simulink model "mpc_aircraft"  (R2015a)
settings: Solver=ode45  SolverMode=SingleTasking  StartTime=0.0  StopTime=10  RelTol=1e-3
values from neighbouring files (symbols this model uses):
  A = [-0.0151 -60.5651 0 -32.174 ... (first row only)    [mpcaircraft.m]
  B = [-2.516 -13.136 ... (first row only)    [mpcaircraft.m]
  C = [0 1 0 0 ... (first row only)    [mpcaircraft.m]
  D = [0 0 ... (first row only)    [mpcaircraft.m]
  p = 10    [mpcaircraft.m]
  x0 = zeros(4,1)    [mpcaircraft.m]
undefined symbols (not defined in the file or in its folder): iA, lastu, lastx, MVscale, nv, nym, Rscale, st, ts, uoff, xoff
libraries: mpcsigdimcheck_private x14
settings Model: CovSFcnEnable=off  ExtModeTrigMode=oneshot  ExtModeArmWhenConnect=off  Creator=The MathWorks Inc.  LastModifiedBy=Yi
settings OptimizationCC: BlockReduction=off  BooleanDataType=off
settings DebuggingCC: SaveWithParameterizedLinksMsg=none  UnderspecifiedInitializationDetection=Classic  MergeDetectMultiDrivingBlocksExec=none  SignalResolutionControl=TryResolveAllWithWarning
settings HardwareCC: TargetUnknown=on

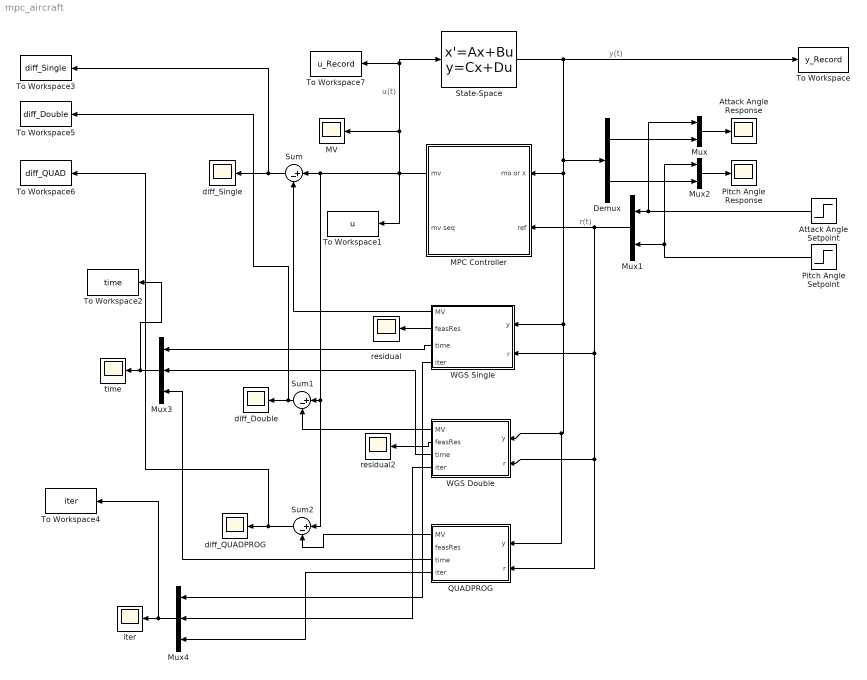
== system mpc_aircraft ==
  note: u(t)
  note: y(t)
  note: r(t)
  Attack Angle Response : Scope
      settings: TimeRange=7  YMin=-0.05  YMax=0.15  DataFormat=Structure
  Attack Angle Setpoint : Step  Time=4  After=0.1  SampleTime=0
  Demux : Demux  Outputs=2
  MPC Controller : Subsystem  AncestorBlock=mpclib/MPC Controller  InitFcn=impcblock_InitFcn  StartFcn=impcblock_StartFcn  mask(MPC){mpcobj=mpcobj, x0=[], is_multiple=0, enable_value=0, n_mv=2, n_mo=2, n_md=0, n_ts=0.05, is_designfromscratch=0, return_u0=off, ref_from_ws=off, ref_signal_name=[], ref_preview=on, md_from_ws=off, md_signal_name=[], md_preview=on, from_project=off, project_file=MPCtask.mat, project_name=, task_name=, md_inport=off, mv_inport=off, cost_outport=off, return_sequence=on, return_qpstatus=off, return_state=off, state_inport=off, lims_inport=off, ywt_inport=off, uwt_inport=off, duwt_inport=off, rhoeps_inport=off, uref_inport=off, BlockDataType=double, SampleTimeInherited=off, switch_inport=off}
      mask prompts: mpcobj "MPC:general:BlgIMPC"; x0 "MPC:general:BlgState"; is_multiple "Flag indicating the block is part of multiple blocks"; enable_value "Value enabling optimization"; n_mv "Number of MVs"; n_mo "Number of MOs"; n_md "Number of MDs"; n_ts "Sample Time"; is_designfromscratch "Design from scratch flag"; return_u0 "Export u0"; ref_from_ws "Obsolete"; ref_signal_name "Obsolete"; ref_preview "Obsolete"; md_from_ws "Obsolete"; md_signal_name "Obsolete"; md_preview "Obsolete"; from_project "Obsolete"; project_file "Obsolete"; project_name "Obsolete"; task_name "Obsolete"; md_inport "MPC:general:BlgMD"; mv_inport "MPC:general:BlgEXTMV"; cost_outport "MPC:general:BlgCOST"; return_sequence "MPC:general:BlgMVSEQ"; return_qpstatus "MPC:general:BlgQPSTATUS"; return_state "MPC:general:BlgESTSTATE"; state_inport "MPC:general:BlgXKK"; lims_inport "MPC:general:BlgLIMITS"; ywt_inport "MPC:general:BlgYWT"; uwt_inport "MPC:general:BlgUWT"; duwt_inport "MPC:general:BlgDUWT"; rhoeps_inport "MPC:general:BlgECRWT"; uref_inport "MPC:general:BlgMVTARGET"; BlockDataType "MPC:general:BlgDATATYPE"; SampleTimeInherited "MPC:general:BlgTS"; switch_inport "MPC:general:BlgSWITCH"
      mask help: MPC:utility:MaskDescMPC1
      mask init:
      | [blk,ts,A,Cm,Bu,Bv,Dvm,isQP,strmoorx,nmoorx,nu,nv,ny,nx,nym...
      |     degrees,L,M,H,Hinv,Linv,iA,Ac,Kx,Ku1,Kut,Kr,Kv,...
      |     Mlim,Mx,Mu1,Mv,z_degrees,utarget,...
      |     lastx,lastu,p,xoff,uoff,yoff,voff,myoff,no_md,no_ref,...
      |     maxiter,nxQP,openloopflag,no_ym,...
      |     lims_inport,no_umin,no_umax,no_ymin,no_ymax,...
      |     switch_inport,no_switch,enable_value,...
      |     return_cost,return_sequence,CustomEstimation,...
      |     no_ywt, no_uwt, no_duwt, no_rhoeps, no_uref, no_mv, ...
      |     Wy,Wdu,Jm,SuJm,Su1,Sx,Hv,Wu,I1,...
      |     isAdaptive, C, Dv, Mrows, nCC, Ecc, Fcc, Scc, Gcc, ...
      |     Uscale, Yscale, nxp, nxindist, mvindex, mdindex, unindex,  ...
      |     myindex,Rscale,MVscale,MDscale] = impcblock_MaskInitFcnParameter();
      | impcblock_MaskInitFcnResize(gcb,nv,nu,ny);
      settings: DeleteFcn=impcblock_DeleteFcn
      mask Help: eval('mpcCSHelp(''MPCmask'',''HelpBrowser'')');
      mask Callback state_inport: mpc_blockdialogcallback(gcb);
      mask DialogControl design_button Prompt: MPC:general:BlgDesignButton
      mask DialogControl design_button Callback: mpc_designcallback(gcbh)
      mask DialogControl review_button Prompt: MPC:general:BlgReviewButton
      mask DialogControl review_button Callback: mpc_reviewcallback(gcbh)
      mask Display:
      | fprintf('MPC');
      | port_label('output', 1, 'mv')
      | port_label('input', 1, 'mo')
      | port_label('input', 2, 'ref')
      | port_label('output', 2, 'mv.seq')
  MV : Scope
      settings: TimeRange=7  YMin=-0.05  YMax=0.15  SaveName=ScopeData11  DataFormat=Structure
  Mux : Mux  Inputs=2
  Mux1 : Mux  Inputs=2
  Mux2 : Mux  Inputs=2
  Mux3 : Mux  Inputs=3
  Mux4 : Mux  Inputs=3
  Pitch Angle Response : Scope
      settings: TimeRange=7  YMin=0  YMax=15  DataFormat=Structure
  Pitch Angle Setpoint : Step  After=10  SampleTime=0
  QUADPROG : Subsystem
  State-Space : StateSpace  A=A  B=B  C=C  D=D  X0=x0
  Sum : Sum  Inputs=|+-
  Sum1 : Sum  Inputs=|+-
  Sum2 : Sum  Inputs=|+-
  To Workspace : ToWorkspace  VariableName=y_Record  SampleTime=-1
  To Workspace1 : ToWorkspace  VariableName=u  SampleTime=-1
  To Workspace2 : ToWorkspace  VariableName=time  SampleTime=-1
  To Workspace3 : ToWorkspace  VariableName=diff_Single  SampleTime=-1
  To Workspace4 : ToWorkspace  VariableName=iter  SampleTime=-1
  To Workspace5 : ToWorkspace  VariableName=diff_Double  SampleTime=-1
  To Workspace6 : ToWorkspace  VariableName=diff_QUAD  SampleTime=-1
  To Workspace7 : ToWorkspace  VariableName=u_Record  SampleTime=-1
  WGS Double : Subsystem
  WGS Single : Subsystem
  diff_Double : Scope
      settings: TimeRange=7  YMin=-0.05  YMax=0.15  SaveName=ScopeData4  DataFormat=Structure
  diff_QUADPROG : Scope
      settings: TimeRange=7  YMin=-0.05  YMax=0.15  SaveName=ScopeData9  DataFormat=Structure
  diff_Single : Scope
      settings: TimeRange=7  YMin=-0.05  YMax=0.15  SaveName=ScopeData3  DataFormat=Structure
  iter : Scope
      settings: TimeRange=7  YMin=-0.05  YMax=0.15  SaveName=ScopeData10  DataFormat=Structure
  residual : Scope
      settings: TimeRange=7  YMin=-0.05  YMax=0.15  SaveName=ScopeData2  DataFormat=Structure
  residual2 : Scope
      settings: TimeRange=7  YMin=-0.05  YMax=0.15  SaveName=ScopeData7  DataFormat=Structure
  "time " : Scope
      settings: TimeRange=7  YMin=-0.05  YMax=0.15  SaveName=ScopeData8  DataFormat=Structure
  wires:
  State-Space/1 -> To Workspace/1, QUADPROG/1(y), WGS Double/1(y), WGS Single/1(y), MPC Controller/1(mo or x), Demux/1
  Mux/1 -> Attack Angle Response/1
  MPC Controller/1(mv) -> MV/1, To Workspace7/1, State-Space/1, Sum2/1, Sum1/1, Sum/1, To Workspace1/1
  Attack Angle Setpoint/1 -> Mux/1, Mux1/1
  Pitch Angle Setpoint/1 -> Mux2/1, Mux1/2
  Mux1/1 -> QUADPROG/2(r), WGS Double/2(r), WGS Single/2(r), MPC Controller/2(ref)
  Demux/1 -> Mux/2
  Mux2/1 -> Pitch Angle Response/1
  Demux/2 -> Mux2/2
  WGS Single/1(MV) -> Sum/2
  WGS Single/2(feasRes) -> residual/1
  WGS Double/1(MV) -> Sum1/2
  WGS Double/2(feasRes) -> residual2/1
  WGS Double/3(time) -> Mux3/2
  Mux3/1 -> To Workspace2/1, "time "/1
  QUADPROG/3(time) -> Mux3/3
  QUADPROG/1(MV) -> Sum2/2
  WGS Single/3(time) -> Mux3/1
  WGS Double/4(iter) -> Mux4/2
  Mux4/1 -> To Workspace4/1, iter/1
  QUADPROG/4(iter) -> Mux4/3
  WGS Single/4(iter) -> Mux4/1
  Sum/1 -> To Workspace3/1, diff_Single/1
  Sum1/1 -> To Workspace5/1, diff_Double/1
  Sum2/1 -> To Workspace6/1, diff_QUADPROG/1

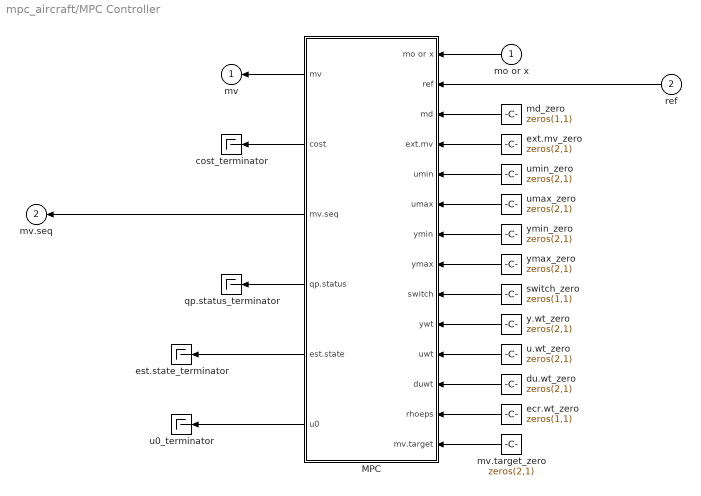
== system mpc_aircraft/MPC Controller ==
  mo or x : Inport
  ref : Inport  Port=2
  MPC : Subsystem
  cost_terminator : Terminator
  du.wt_zero : Constant  Value=zeros(2,1)  OutDataTypeStr=BlockDataType
  ecr.wt_zero : Constant  Value=zeros(1,1)  OutDataTypeStr=BlockDataType
  est.state_terminator : Terminator
  ext.mv_zero : Constant  Value=zeros(2,1)  OutDataTypeStr=BlockDataType
  md_zero : Constant  Value=zeros(1,1)  OutDataTypeStr=BlockDataType
  mv.target_zero : Constant  Value=zeros(2,1)  OutDataTypeStr=BlockDataType
  qp.status_terminator : Terminator
  switch_zero : Constant  Value=zeros(1,1)  OutDataTypeStr=BlockDataType
  u.wt_zero : Constant  Value=zeros(2,1)  OutDataTypeStr=BlockDataType
  u0_terminator : Terminator
  umax_zero : Constant  Value=zeros(2,1)  OutDataTypeStr=BlockDataType
  umin_zero : Constant  Value=zeros(2,1)  OutDataTypeStr=BlockDataType
  y.wt_zero : Constant  Value=zeros(2,1)  OutDataTypeStr=BlockDataType
  ymax_zero : Constant  Value=zeros(2,1)  OutDataTypeStr=BlockDataType
  ymin_zero : Constant  Value=zeros(2,1)  OutDataTypeStr=BlockDataType
  mv : Outport
  mv.seq : Outport  Port=2
  wires:
  ext.mv_zero/1 -> MPC/4(ext.mv)
  MPC/5(est.state) -> est.state_terminator/1
  MPC/6(u0) -> u0_terminator/1
  ymax_zero/1 -> MPC/8(ymax)
  ymin_zero/1 -> MPC/7(ymin)
  umax_zero/1 -> MPC/6(umax)
  umin_zero/1 -> MPC/5(umin)
  switch_zero/1 -> MPC/9(switch)
  mv.target_zero/1 -> MPC/14(mv.target)
  u.wt_zero/1 -> MPC/11(uwt)
  MPC/4(qp.status) -> qp.status_terminator/1
  MPC/2(cost) -> cost_terminator/1
  ecr.wt_zero/1 -> MPC/13(rhoeps)
  du.wt_zero/1 -> MPC/12(duwt)
  y.wt_zero/1 -> MPC/10(ywt)
  MPC/1(mv) -> mv/1
  mo or x/1 -> MPC/1(mo or x)
  ref/1 -> MPC/2(ref)
  md_zero/1 -> MPC/3(md)
  MPC/3(mv.seq) -> mv.seq/1

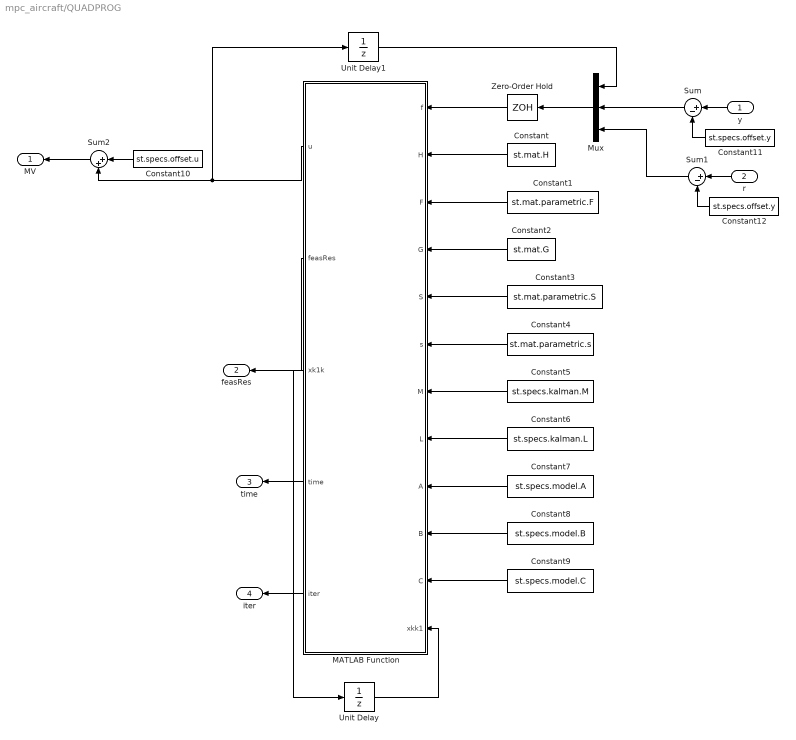
== system mpc_aircraft/QUADPROG ==
  y : Inport
  r : Inport  Port=2
  Constant : Constant  Value=st.mat.H
  Constant1 : Constant  Value=st.mat.parametric.F
  Constant10 : Constant  Value=st.specs.offset.u
  Constant11 : Constant  Value=st.specs.offset.y
  Constant12 : Constant  Value=st.specs.offset.y
  Constant2 : Constant  Value=st.mat.G
  Constant3 : Constant  Value=st.mat.parametric.S
  Constant4 : Constant  Value=st.mat.parametric.s
  Constant5 : Constant  Value=st.specs.kalman.M
  Constant6 : Constant  Value=st.specs.kalman.L
  Constant7 : Constant  Value=st.specs.model.A
  Constant8 : Constant  Value=st.specs.model.B
  Constant9 : Constant  Value=st.specs.model.C
  MATLAB Function : MATLAB Function  TreatAsAtomicUnit=on
  Mux : Mux  Inputs=3
  Sum : Sum  Inputs=|+-
  Sum1 : Sum  Inputs=|+-
  Sum2 : Sum  Inputs=|++
  Unit Delay : UnitDelay  InitialCondition=st.specs.init.x0  SampleTime=st.specs.model.Ts
  Unit Delay1 : UnitDelay  InitialCondition=st.specs.init.u0  SampleTime=st.specs.model.Ts
  Zero-Order Hold : ZeroOrderHold  SampleTime=st.specs.model.Ts
  MV : Outport
  feasRes : Outport  Port=2
  time : Outport  Port=3
  iter : Outport  Port=4
  wires:
  Sum2/1 -> MV/1
  Constant10/1 -> Sum2/1
  r/1 -> Sum1/1
  Sum1/1 -> Mux/3
  Constant12/1 -> Sum1/2
  y/1 -> Sum/1
  Sum/1 -> Mux/2
  Constant11/1 -> Sum/2
  Unit Delay1/1 -> Mux/1
  Mux/1 -> Zero-Order Hold/1
  MATLAB Function/2(feasRes) -> feasRes/1
  Constant9/1 -> MATLAB Function/11(C)
  MATLAB Function/3(xk1k) -> Unit Delay/1
  Zero-Order Hold/1 -> MATLAB Function/1(f)
  Constant/1 -> MATLAB Function/2(H)
  Constant1/1 -> MATLAB Function/3(F)
  Constant2/1 -> MATLAB Function/4(G)
  Constant3/1 -> MATLAB Function/5(S)
  Constant4/1 -> MATLAB Function/6(s)
  Constant5/1 -> MATLAB Function/7(M)
  Constant6/1 -> MATLAB Function/8(L)
  Constant7/1 -> MATLAB Function/9(A)
  Constant8/1 -> MATLAB Function/10(B)
  MATLAB Function/1(u) -> Sum2/2, Unit Delay1/1
  Unit Delay/1 -> MATLAB Function/12(xkk1)
  MATLAB Function/4(time) -> time/1
  MATLAB Function/5(iter) -> iter/1

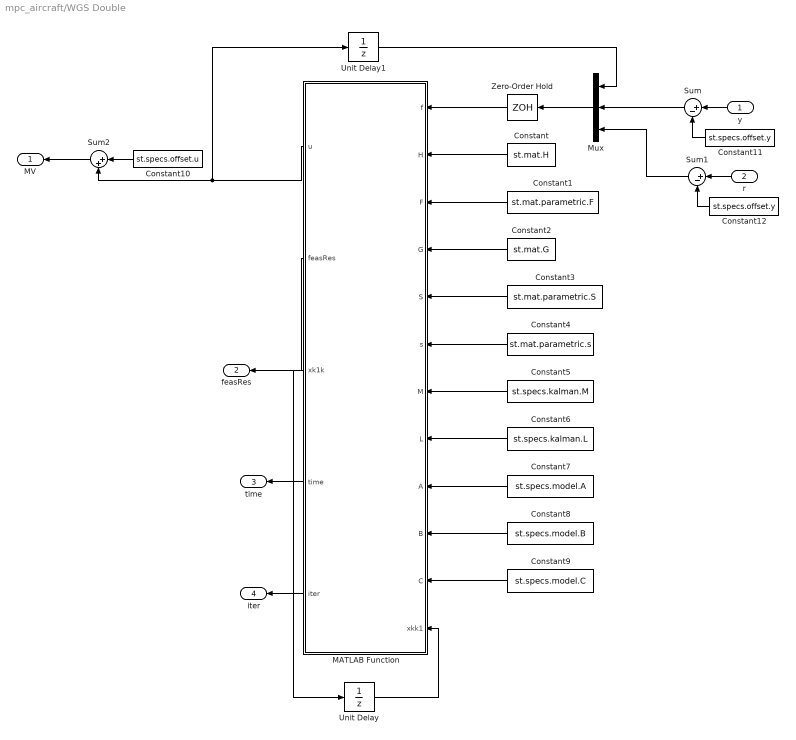
== system mpc_aircraft/WGS Double ==
  y : Inport
  r : Inport  Port=2
  Constant : Constant  Value=st.mat.H
  Constant1 : Constant  Value=st.mat.parametric.F
  Constant10 : Constant  Value=st.specs.offset.u
  Constant11 : Constant  Value=st.specs.offset.y
  Constant12 : Constant  Value=st.specs.offset.y
  Constant2 : Constant  Value=st.mat.G
  Constant3 : Constant  Value=st.mat.parametric.S
  Constant4 : Constant  Value=st.mat.parametric.s
  Constant5 : Constant  Value=st.specs.kalman.M
  Constant6 : Constant  Value=st.specs.kalman.L
  Constant7 : Constant  Value=st.specs.model.A
  Constant8 : Constant  Value=st.specs.model.B
  Constant9 : Constant  Value=st.specs.model.C
  MATLAB Function : MATLAB Function  TreatAsAtomicUnit=on
  Mux : Mux  Inputs=3
  Sum : Sum  Inputs=|+-
  Sum1 : Sum  Inputs=|+-
  Sum2 : Sum  Inputs=|++
  Unit Delay : UnitDelay  InitialCondition=st.specs.init.x0  SampleTime=st.specs.model.Ts
  Unit Delay1 : UnitDelay  InitialCondition=st.specs.init.u0  SampleTime=st.specs.model.Ts
  Zero-Order Hold : ZeroOrderHold  SampleTime=st.specs.model.Ts
  MV : Outport
  feasRes : Outport  Port=2
  time : Outport  Port=3
  iter : Outport  Port=4
  wires:
  Sum2/1 -> MV/1
  Constant10/1 -> Sum2/1
  r/1 -> Sum1/1
  Sum1/1 -> Mux/3
  Constant12/1 -> Sum1/2
  y/1 -> Sum/1
  Sum/1 -> Mux/2
  Constant11/1 -> Sum/2
  Unit Delay1/1 -> Mux/1
  Mux/1 -> Zero-Order Hold/1
  MATLAB Function/2(feasRes) -> feasRes/1
  Constant9/1 -> MATLAB Function/11(C)
  MATLAB Function/3(xk1k) -> Unit Delay/1
  Zero-Order Hold/1 -> MATLAB Function/1(f)
  Constant/1 -> MATLAB Function/2(H)
  Constant1/1 -> MATLAB Function/3(F)
  Constant2/1 -> MATLAB Function/4(G)
  Constant3/1 -> MATLAB Function/5(S)
  Constant4/1 -> MATLAB Function/6(s)
  Constant5/1 -> MATLAB Function/7(M)
  Constant6/1 -> MATLAB Function/8(L)
  Constant7/1 -> MATLAB Function/9(A)
  Constant8/1 -> MATLAB Function/10(B)
  MATLAB Function/1(u) -> Sum2/2, Unit Delay1/1
  Unit Delay/1 -> MATLAB Function/12(xkk1)
  MATLAB Function/4(time) -> time/1
  MATLAB Function/5(iter) -> iter/1

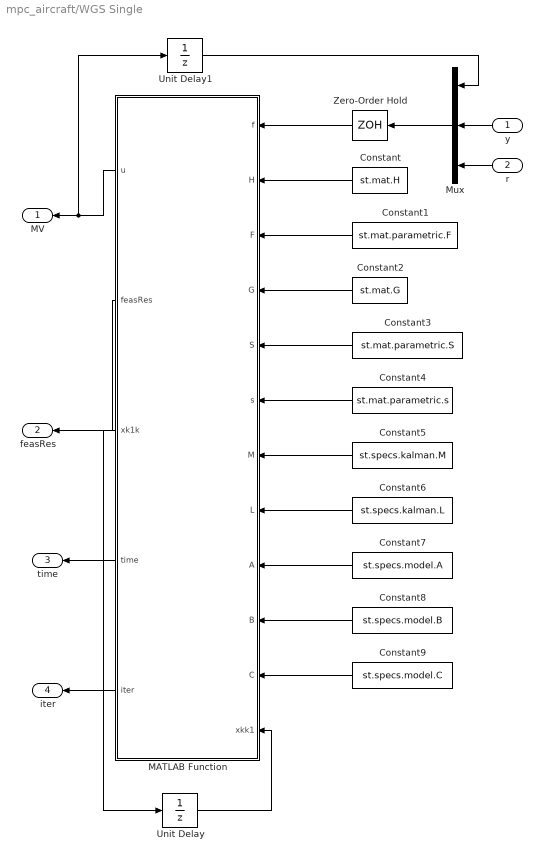
== system mpc_aircraft/WGS Single ==
  y : Inport
  r : Inport  Port=2
  Constant : Constant  Value=st.mat.H
  Constant1 : Constant  Value=st.mat.parametric.F
  Constant2 : Constant  Value=st.mat.G
  Constant3 : Constant  Value=st.mat.parametric.S
  Constant4 : Constant  Value=st.mat.parametric.s
  Constant5 : Constant  Value=st.specs.kalman.M
  Constant6 : Constant  Value=st.specs.kalman.L
  Constant7 : Constant  Value=st.specs.model.A
  Constant8 : Constant  Value=st.specs.model.B
  Constant9 : Constant  Value=st.specs.model.C
  MATLAB Function : MATLAB Function  TreatAsAtomicUnit=on
  Mux : Mux  Inputs=3
  Unit Delay : UnitDelay  InitialCondition=st.specs.init.x0  SampleTime=st.specs.model.Ts
  Unit Delay1 : UnitDelay  InitialCondition=st.specs.init.u0  SampleTime=st.specs.model.Ts
  Zero-Order Hold : ZeroOrderHold  SampleTime=st.specs.model.Ts
  MV : Outport
  feasRes : Outport  Port=2
  time : Outport  Port=3
  iter : Outport  Port=4
  wires:
  Zero-Order Hold/1 -> MATLAB Function/1(f)
  Unit Delay/1 -> MATLAB Function/12(xkk1)
  MATLAB Function/3(xk1k) -> Unit Delay/1
  Constant9/1 -> MATLAB Function/11(C)
  Constant8/1 -> MATLAB Function/10(B)
  Constant7/1 -> MATLAB Function/9(A)
  Constant6/1 -> MATLAB Function/8(L)
  Constant5/1 -> MATLAB Function/7(M)
  MATLAB Function/2(feasRes) -> feasRes/1
  Constant4/1 -> MATLAB Function/6(s)
  Constant3/1 -> MATLAB Function/5(S)
  Constant2/1 -> MATLAB Function/4(G)
  Constant1/1 -> MATLAB Function/3(F)
  Constant/1 -> MATLAB Function/2(H)
  Mux/1 -> Zero-Order Hold/1
  r/1 -> Mux/3
  y/1 -> Mux/2
  Unit Delay1/1 -> Mux/1
  MATLAB Function/1(u) -> MV/1, Unit Delay1/1
  MATLAB Function/4(time) -> time/1
  MATLAB Function/5(iter) -> iter/1

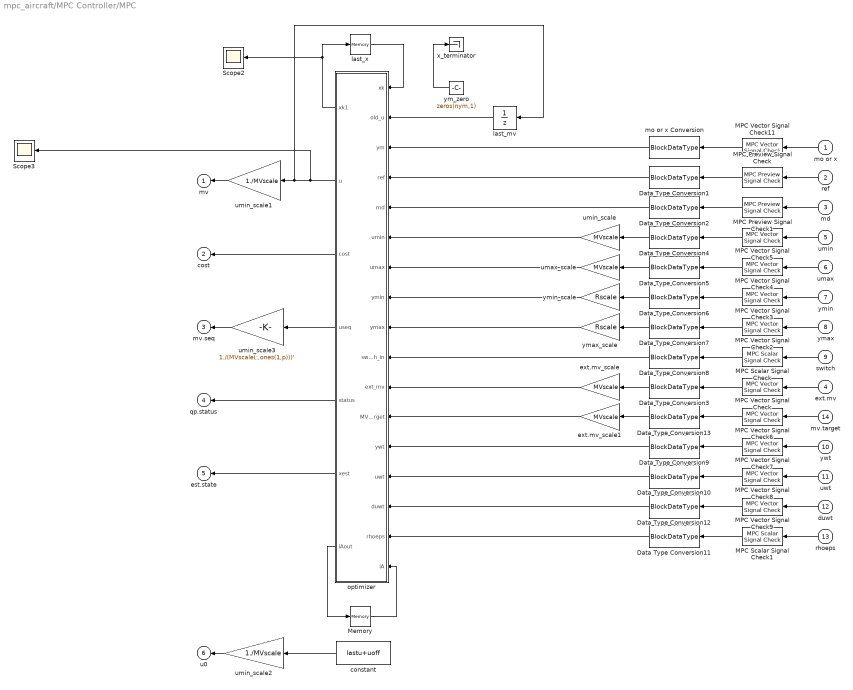
== system mpc_aircraft/MPC Controller/MPC ==
  mo or x : Inport
  ref : Inport  Port=2
  md : Inport  Port=3
  ext.mv : Inport  Port=4
  umin : Inport  Port=5
  umax : Inport  Port=6
  ymin : Inport  Port=7
  ymax : Inport  Port=8
  switch : Inport  Port=9
  ywt : Inport  Port=10
  uwt : Inport  Port=11
  duwt : Inport  Port=12
  rhoeps : Inport  Port=13
  mv.target : Inport  Port=14
  Data Type Conversion{1..13} (13 alike) : DataTypeConversion  OutDataTypeStr=BlockDataType
  MPC Preview Signal Check : mpcsigdimcheck_private/MPC Preview Signal Check  blockname=blk  signalname='ref'  numrow=p  numcol=ny
  MPC Preview Signal Check1 : mpcsigdimcheck_private/MPC Preview Signal Check  blockname=blk  signalname='md'  numrow=p+1  numcol=max(nv-1,1)
  MPC Scalar Signal Check : mpcsigdimcheck_private/MPC Scalar Signal Check  blockname=blk  signalname='switch'
  MPC Scalar Signal Check1 : mpcsigdimcheck_private/MPC Scalar Signal Check  blockname=blk  signalname='ecr.wt'
  MPC Vector Signal Check : mpcsigdimcheck_private/MPC Vector Signal Check  blockname=blk  signalname='ext.mv'  num=nu  vectortype=Any
  MPC Vector Signal Check11 : mpcsigdimcheck_private/MPC Vector Signal Check  blockname=blk  signalname=strmoorx  num=nmoorx  vectortype=Any
  MPC Vector Signal Check2 : mpcsigdimcheck_private/MPC Vector Signal Check  blockname=blk  signalname='ymax'  num=ny  vectortype=Any
  MPC Vector Signal Check3 : mpcsigdimcheck_private/MPC Vector Signal Check  blockname=blk  signalname='ymin'  num=ny  vectortype=Any
  MPC Vector Signal Check4 : mpcsigdimcheck_private/MPC Vector Signal Check  blockname=blk  signalname='umax'  num=nu  vectortype=Any
  MPC Vector Signal Check5 : mpcsigdimcheck_private/MPC Vector Signal Check  blockname=blk  signalname='umin'  num=nu  vectortype=Any
  MPC Vector Signal Check6 : mpcsigdimcheck_private/MPC Vector Signal Check  blockname=blk  signalname='mv.target'  num=nu  vectortype=Any
  MPC Vector Signal Check7 : mpcsigdimcheck_private/MPC Vector Signal Check  blockname=blk  signalname='y.wt'  num=ny  vectortype=Any
  MPC Vector Signal Check8 : mpcsigdimcheck_private/MPC Vector Signal Check  blockname=blk  signalname='u.wt'  num=nu  vectortype=Any
  MPC Vector Signal Check9 : mpcsigdimcheck_private/MPC Vector Signal Check  blockname=blk  signalname='du.wt'  num=nu  vectortype=Any
  Memory : Memory  X0=iA  InheritSampleTime=on  LinearizeAsDelay=on
  Scope2 : Scope
      settings: SaveName=ScopeData5
  Scope3 : Scope
      settings: SaveName=ScopeData6
  constant : Constant  Value=lastu+uoff
  ext.mv_scale : Gain  Gain=MVscale  SampleTime=ts
  ext.mv_scale1 : Gain  Gain=MVscale  SampleTime=ts
  last_mv : UnitDelay  InitialCondition=lastu+uoff  SampleTime=ts
  last_x : Memory  X0=lastx+xoff  InheritSampleTime=on  LinearizeAsDelay=on
  mo or x Conversion : DataTypeConversion  OutDataTypeStr=BlockDataType
  optimizer : MATLAB Function
  umax_scale : Gain  Gain=MVscale  SampleTime=ts
  umin_scale : Gain  Gain=MVscale  SampleTime=ts
  umin_scale1 : Gain  Gain=1./MVscale  SampleTime=ts
  umin_scale2 : Gain  Gain=1./MVscale  SampleTime=ts
  umin_scale3 : Gain  Gain=1./(MVscale(:,ones(1,p)))'  SampleTime=ts
  x_terminator : Terminator
  ym_zero : Constant  Value=zeros(nym,1)  OutDataTypeStr=BlockDataType
  ymax_scale : Gain  Gain=Rscale  SampleTime=ts
  ymin_scale : Gain  Gain=Rscale  SampleTime=ts
  mv : Outport  OutDataTypeStr=BlockDataType
  cost : Outport  Port=2  OutDataTypeStr=BlockDataType
  mv.seq : Outport  Port=3  OutDataTypeStr=BlockDataType
  qp.status : Outport  Port=4  OutDataTypeStr=BlockDataType
  est.state : Outport  Port=5  OutDataTypeStr=BlockDataType
  u0 : Outport  Port=6  OutDataTypeStr=BlockDataType
  wires:
  MPC Preview Signal Check1/1 -> Data Type Conversion2/1
  MPC Preview Signal Check/1 -> Data Type Conversion1/1
  MPC Vector Signal Check11/1 -> mo or x Conversion/1
  MPC Scalar Signal Check1/1 -> Data Type Conversion11/1
  MPC Vector Signal Check9/1 -> Data Type Conversion12/1
  MPC Vector Signal Check8/1 -> Data Type Conversion10/1
  MPC Vector Signal Check7/1 -> Data Type Conversion9/1
  MPC Vector Signal Check6/1 -> Data Type Conversion13/1
  MPC Vector Signal Check5/1 -> Data Type Conversion4/1
  MPC Vector Signal Check4/1 -> Data Type Conversion5/1
  MPC Vector Signal Check3/1 -> Data Type Conversion6/1
  MPC Vector Signal Check2/1 -> Data Type Conversion7/1
  MPC Scalar Signal Check/1 -> Data Type Conversion8/1
  MPC Vector Signal Check/1 -> Data Type Conversion3/1
  ym_zero/1 -> x_terminator/1
  mo or x Conversion/1 -> optimizer/3(ym)
  optimizer/6(xest) -> est.state/1
  umin_scale3/1 -> mv.seq/1
  umin_scale1/1 -> mv/1
  umin_scale2/1 -> u0/1
  constant/1 -> umin_scale2/1
  ext.mv_scale/1 -> optimizer/11(ext_mv)
  optimizer/2(u) -> Scope3/1, umin_scale1/1, last_mv/1
  Data Type Conversion1/1 -> optimizer/4(ref)
  ext.mv_scale1/1 -> optimizer/12(MVtarget)
  Data Type Conversion13/1 -> ext.mv_scale1/1
  mv.target/1 -> MPC Vector Signal Check6/1
  optimizer/1(xk1) -> Scope2/1, last_x/1
  Data Type Conversion10/1 -> optimizer/14(uwt)
  duwt/1 -> MPC Vector Signal Check9/1
  rhoeps/1 -> MPC Scalar Signal Check1/1
  Data Type Conversion2/1 -> optimizer/5(md)
  ymax_scale/1 -> optimizer/9(ymax)
  ymin_scale/1 -> optimizer/8(ymin)
  Data Type Conversion6/1 -> ymin_scale/1
  umax_scale/1 -> optimizer/7(umax)
  umin_scale/1 -> optimizer/6(umin)
  Data Type Conversion11/1 -> optimizer/16(rhoeps)
  Data Type Conversion12/1 -> optimizer/15(duwt)
  Data Type Conversion9/1 -> optimizer/13(ywt)
  Data Type Conversion8/1 -> optimizer/10(switch_in)
  Data Type Conversion7/1 -> ymax_scale/1
  Data Type Conversion5/1 -> umax_scale/1
  Data Type Conversion4/1 -> umin_scale/1
  uwt/1 -> MPC Vector Signal Check8/1
  ywt/1 -> MPC Vector Signal Check7/1
  optimizer/7(iAout) -> Memory/1
  optimizer/5(status) -> qp.status/1
  Memory/1 -> optimizer/17(iA)
  mo or x/1 -> MPC Vector Signal Check11/1
  ref/1 -> MPC Preview Signal Check/1
  last_mv/1 -> optimizer/2(old_u)
  Data Type Conversion3/1 -> ext.mv_scale/1
  ext.mv/1 -> MPC Vector Signal Check/1
  switch/1 -> MPC Scalar Signal Check/1
  ymax/1 -> MPC Vector Signal Check2/1
  ymin/1 -> MPC Vector Signal Check3/1
  umax/1 -> MPC Vector Signal Check4/1
  umin/1 -> MPC Vector Signal Check5/1
  md/1 -> MPC Preview Signal Check1/1
  optimizer/3(cost) -> cost/1
  optimizer/4(useq) -> umin_scale3/1
  last_x/1 -> optimizer/1(xk)

== matlab function mpc_aircraft/WGS Single/MATLAB Function ==
  data: f input; H input; F input; G input; S input; s input; u output; feasRes output; M input; L input; xk1k output; A input; B input; C input; xkk1 input; time output; iter output
%% solve the problem
%   min 0.5 z'Hz + h'z
%   s.t. Gz <= b

function [u,feasRes,xk1k,time,iter]=fcn(f,H,F,G,S,s,M,L,A,B,C,xkk1)
%% init
coder.extrinsic('quadprog');
coder.extrinsic('wgsSolver');

options.Algorithm='interior-point-convex';
options.MaxIter=1000;
options.TolCon=1.0000e-12; % default: 1e-8
options.TolFun=1.0000e-12; % default: 1e-8
options.TolX=1.0000e-12;   % default: 1e-8
options.Display='none';
zopt=zeros(size(H,1),1);
time = 0;
iter = 0;

%% get info
[~,nu]=size(B);
ny=size(C,1);
u0=f(1:nu);
y=f(nu+1:nu+ny);

xkk=xkk1+M*(y-C*xkk1);  % kalman

%% solver
p=[f(1:nu);xkk;f(ny+nu+1:2*ny+nu)];

b=S*p+s;
h=F*p;
%[zopt]=quadprog(H,h,G,b,[],[],[],[],[],options); % solve the optimal control problem
[zopt,time,iter] = wgsSolver(H,h,-G,-b,[],[],[],[],[],1);


feasRes=G*zopt-b;

nu=length(u0);
u=zopt(1:nu)+u0;

xk1k=A*xkk1+B*u+L*(y-C*xkk1); % kalman

== matlab function mpc_aircraft/WGS Double/MATLAB Function ==
  data: f input; H input; F input; G input; S input; s input; u output; feasRes output; M input; L input; xk1k output; A input; B input; C input; xkk1 input; time output; iter output
%% solve the problem
%   min 0.5 z'Hz + h'z
%   s.t. Gz <= b

function [u,feasRes,xk1k,time,iter]=fcn(f,H,F,G,S,s,M,L,A,B,C,xkk1)
%% init
coder.extrinsic('quadprog');
coder.extrinsic('wgsSolver');
options.Algorithm='interior-point-convex';
options.MaxIter=1000;
options.TolCon=1.0000e-12; % default: 1e-8
options.TolFun=1.0000e-12; % default: 1e-8
options.TolX=1.0000e-12;   % default: 1e-8
options.Display='none';
zopt=zeros(size(H,1),1);
time = 0;
iter = 0;

%% get info
[~,nu]=size(B);
ny=size(C,1);
u0=f(1:nu);
y=f(nu+1:nu+ny);

xkk=xkk1+M*(y-C*xkk1);  % kalman

%% solver
p=[f(1:nu);xkk;f(ny+nu+1:2*ny+nu)];

b=S*p+s;
h=F*p;
%[zopt]=quadprog(H,h,G,b,[],[],[],[],[],options); % solve the optimal control problem
[zopt,time,iter] = wgsSolver(H,h,-G,-b,[],[],[],[],[],2);    % first goldfarb
feasRes=G*zopt-b;

nu=length(u0);
u=zopt(1:nu)+u0;

xk1k=A*xkk1+B*u+L*(y-C*xkk1); % kalman

== matlab function mpc_aircraft/MPC Controller/MPC/optimizer ==
  settings: updateMethod=DISCRETE  sampleTime=ts
  data: xk1 output BlockDataType; xk input BlockDataType; old_u input BlockDataType; ym input BlockDataType; ref input BlockDataType; md input BlockDataType; umin input BlockDataType; umax input BlockDataType; ymin input BlockDataType; ymax input BlockDataType; switch_in input BlockDataType; ext_mv input BlockDataType; MVtarget input BlockDataType; isQP parameter boolean; nx parameter BlockDataType; nu parameter BlockDataType; ny parameter BlockDataType; degrees parameter BlockDataType; Hinv parameter BlockDataType; Kx parameter BlockDataType; Ku1 parameter BlockDataType; Kut parameter BlockDataType; Kr parameter BlockDataType; Kv parameter BlockDataType; Mlim parameter BlockDataType; Mx parameter BlockDataType; Mu1 parameter BlockDataType; Mv parameter BlockDataType; z_degrees parameter BlockDataType; utarget parameter BlockDataType; p parameter BlockDataType; uoff parameter BlockDataType; voff parameter BlockDataType; yoff parameter BlockDataType; maxiter parameter BlockDataType; nxQP parameter BlockDataType; openloopflag parameter boolean; lims_inport parameter BlockDataType; no_umin parameter BlockDataType; no_umax parameter BlockDataType; no_ymin parameter BlockDataType; no_ymax parameter BlockDataType; switch_inport parameter BlockDataType; no_switch parameter BlockDataType; enable_value parameter BlockDataType; return_cost parameter BlockDataType; H parameter BlockDataType; return_sequence parameter BlockDataType; Linv parameter BlockDataType; Ac parameter BlockDataType; ywt input BlockDataType; uwt input BlockDataType; duwt input BlockDataType; rhoeps input BlockDataType; iA input boolean; u output BlockDataType; cost output BlockDataType; useq output BlockDataType; status output BlockDataType; xest output BlockDataType; no_ywt parameter BlockDataType; no_uwt parameter BlockDataType; no_duwt parameter BlockDataType; no_rhoeps parameter BlockDataType; Wy parameter BlockDataType; Wdu parameter BlockDataType; Jm parameter BlockDataType; SuJm parameter BlockDataType; Su1 parameter BlockDataType; Sx parameter BlockDataType; Hv parameter BlockDataType; Wu parameter BlockDataType; I1 parameter BlockDataType; iAout output boolean; A parameter BlockDataType; Bu parameter BlockDataType; Bv parameter BlockDataType; C parameter BlockDataType; Dv parameter BlockDataType; Mrows parameter BlockDataType; nCC parameter BlockDataType; Ecc parameter BlockDataType; Fcc parameter BlockDataType; Scc parameter BlockDataType; Gcc parameter BlockDataType; nv parameter BlockDataType; no_md parameter BlockDataType; no_ref parameter BlockDataType; no_uref parameter BlockDataType; no_mv parameter BlockDataType; Rscale parameter BlockDataType; MDscale parameter BlockDataType; myindex parameter BlockDataType; myoff parameter BlockDataType; xoff parameter BlockDataType; CustomEstimation parameter BlockDataType; M parameter BlockDataType; L parameter BlockDataType
function [xk1, u, cost, useq, status, xest, iAout] = fcn(...
            xk, old_u, ym, ref, md, umin, umax, ymin, ymax, switch_in, ext_mv, MVtarget, isQP, nx, nu, ny, degrees, Hinv, Kx, Ku1, Kut, Kr, Kv, Mlim, ...
            Mx, Mu1, Mv, z_degrees, utarget, p, uoff, voff, yoff, maxiter, nxQP, openloopflag, ...
            lims_inport, no_umin, no_umax, no_ymin, no_ymax, switch_inport, no_switch, enable_value, ...
            return_cost, H, return_sequence, Linv, Ac, ...
            ywt, uwt, duwt, rhoeps, iA, ...
            no_ywt, no_uwt, no_duwt, no_rhoeps,...
            Wy, Wdu, Jm, SuJm, Su1, Sx, Hv, Wu, I1, ...
            A, Bu, Bv, C, Dv, Mrows, nCC, Ecc, Fcc, Scc, Gcc, ...
            nv, no_md, no_ref, no_uref, no_mv, Rscale, MDscale, myindex, ...
            myoff, xoff, CustomEstimation, M, L)
%#codegen
coder.extrinsic('mpcblock_optimizer_double_mex');
coder.extrinsic('mpcblock_optimizer_single_mex');
coder.extrinsic('mpcblock_refmd_double_mex');
coder.extrinsic('mpcblock_refmd_single_mex');

% Parameters
isSimulation = coder.target('Sfun') && ~coder.target('RtwForRapid') && ~coder.target('RtwForSim');
isAdaptive = false;
isDouble = isa(ref,'double');
ZERO = zeros('like',ref);
ONE = ones('like',ref);

% Pre-allocate all the MEX block outputs for the simulation mode
%#ok<*NASGU>
%#ok<*PREALL>
if isSimulation
    rseq = zeros(p*ny,1,'like',ref); 
    vseq = zeros((p+1)*nv,1,'like',ref);
    v = zeros(nv,1,'like',ref);
    xk1 = zeros(nx,1,'like',ref);
    u = zeros(nu,1,'like',ref);
    cost =  ZERO;
    useq = zeros(p,nu,'like',ref); 
    status = ONE;
    xest = zeros(nx,1,'like',ref);
    iAout = iA;    
end

% Get reference and MD signals -- accounting for previewing
if isSimulation
    % When doing normal simulation in SL, use MEX for better compilation speed 
    if isDouble
        [rseq, vseq, v] = mpcblock_refmd_double_mex(ref,md,nv,ny,p,yoff,voff,no_md,no_ref,openloopflag, Rscale, MDscale);
    else
        [rseq, vseq, v] = mpcblock_refmd_single_mex(ref,md,nv,ny,p,yoff,voff,no_md,no_ref,openloopflag, Rscale, MDscale);        
    end
else
    % When doing code generation, use M code directly
    [rseq, vseq, v] = mpcblock_refmd(ref,md,nv,ny,p,yoff,voff,no_md,no_ref,openloopflag, Rscale, MDscale);
end

% External MV override.  
% NOTE: old_u and ext_mv input signals are dimensionless but include offset
old_u = old_u - uoff;
if no_mv==ONE
    delmv = zeros(nu,1,'like',ref);
else
    ext_mv = ext_mv - uoff;     % Bias correction
    delmv = ext_mv - old_u;
    old_u = ext_mv;
end

% Obtain x[k|k]
xk = xk - xoff; % Remove offset
if CustomEstimation==ONE
    % Input state is x(k|k)
    xest = xk(:);
else
    % Default state estimation.    
    % Scale measured output and remove offset.
    ym = ym.*Rscale(myindex) - myoff;
    % Correct x(k|k-1) for possible external mv override.
    % NOTE:  Offset was removed from x[k|k-1] at k=0.
    xk = xk + Bu*delmv;
    % Measurement upate to x(k|k)
    ym_est = C(myindex,:)*xk + Dv(myindex,:)*v;
    y_innov = ym - ym_est;
    xest = xk + M*y_innov;
end

% Real-time MV target override
% Note: utargetValue is a vector length p*nu.  
if no_uref==ONE
    % no external utarget
    utargetValue = utarget;
else
    % utarget is a vector length p*nu.  Define constant targets for the
    % entire horizon.
    MVtarget = MVtarget - uoff;         % Bias correction
    utargetValue = reshape(MVtarget(:,ones(p,1)),nu*p,1);
end

if isSimulation
    % When doing normal simulation in SL, use MEX for better compilation speed 
    if isDouble
        [u, cost, useq, status, iAout] = mpcblock_optimizer_double_mex(...
            rseq, vseq, umin, umax, ymin, ymax, switch_in, xest, old_u, iA, ...
            isQP, nu, ny, degrees, Hinv, Kx, Ku1, Kut, Kr, Kv, Mlim, ...
            Mx, Mu1, Mv, z_degrees, utargetValue, p, uoff, voff, yoff, maxiter, nxQP, openloopflag, ...
            lims_inport, no_umin, no_umax, no_ymin, no_ymax, switch_inport, ...
            no_switch, enable_value, return_cost, H, return_sequence, Linv, Ac, ...
            ywt, uwt, duwt, rhoeps, no_ywt, no_uwt, no_duwt, no_rhoeps,...
            Wy, Wdu, Jm, SuJm, Su1, Sx, Hv, Wu, I1, ...
            isAdaptive, A, Bu, Bv, C, Dv, ...
            Mrows, nCC, Ecc, Fcc, Scc, Gcc);    
    else
        [u, cost, useq, status, iAout] = mpcblock_optimizer_single_mex(...
            rseq, vseq, umin, umax, ymin, ymax, switch_in, xest, old_u, iA, ...
            isQP, nu, ny, degrees, Hinv, Kx, Ku1, Kut, Kr, Kv, Mlim, ...
            Mx, Mu1, Mv, z_degrees, utargetValue, p, uoff, voff, yoff, maxiter, nxQP, openloopflag, ...
            lims_inport, no_umin, no_umax, no_ymin, no_ymax, switch_inport, ...
            no_switch, enable_value, return_cost, H, return_sequence, Linv, Ac, ...
            ywt, uwt, duwt, rhoeps, no_ywt, no_uwt, no_duwt, no_rhoeps,...
            Wy, Wdu, Jm, SuJm, Su1, Sx, Hv, Wu, I1, ...
            isAdaptive, A, Bu, Bv, C, Dv, ...
            Mrows, nCC, Ecc, Fcc, Scc, Gcc);    
    end
else
    % When doing code generation, use M code directly
        [u, cost, useq, status, iAout] = mpcblock_optimizer(...
            rseq, vseq, umin, umax, ymin, ymax, switch_in, xest, old_u, iA, ...
            isQP, nu, ny, degrees, Hinv, Kx, Ku1, Kut, Kr, Kv, Mlim, ...
            Mx, Mu1, Mv, z_degrees, utargetValue, p, uoff, voff, yoff, maxiter, nxQP, openloopflag, ...
            lims_inport, no_umin, no_umax, no_ymin, no_ymax, switch_inport, ...
            no_switch, enable_value, return_cost, H, return_sequence, Linv, Ac, ...
            ywt, uwt, duwt, rhoeps, no_ywt, no_uwt, no_duwt, no_rhoeps,...
            Wy, Wdu, Jm, SuJm, Su1, Sx, Hv, Wu, I1, ...
            isAdaptive, A, Bu, Bv, C, Dv, ...
            Mrows, nCC, Ecc, Fcc, Scc, Gcc);    
end

if CustomEstimation==ONE
    xk1 = xk;
else
    % update x[k+1|k], assuming that above u and v will be applied.
    xk1 = A*xk + Bu*(u - uoff) + Bv*v + L*y_innov; 
end
xk1 = xk1 + xoff;   % Updated state must include offset

if CustomEstimation==ONE
    % sent to terminal
    xest = zeros(nx,1,'like',ref);
else
    xest = xest + xoff;
end

== matlab function mpc_aircraft/QUADPROG/MATLAB Function ==
  data: f input; H input; F input; G input; S input; s input; u output; feasRes output; M input; L input; xk1k output; A input; B input; C input; xkk1 input; time output; iter output
%% solve the problem
%   min 0.5 z'Hz + h'z
%   s.t. Gz <= b

function [u,feasRes,xk1k,time,iter]=fcn(f,H,F,G,S,s,M,L,A,B,C,xkk1)
%% init
coder.extrinsic('tic');
coder.extrinsic('toc');
coder.extrinsic('quadprog');
coder.extrinsic('wgsSolver');
options.Algorithm='interior-point-convex';
options.MaxIter=1000;
options.TolCon=1.0000e-12; % default: 1e-8
options.TolFun=1.0000e-12; % default: 1e-8
options.TolX=1.0000e-12;   % default: 1e-8
options.Display='none';
zopt=zeros(size(H,1),1);
time = 0;
iter = 0;
mess = zeros(1,912);
mess = char(mess);
output.message = mess;
output.algorithm = 'interior-point-convex';
output.firstorderopt = 0;
output.constrviolation = 0;
output.iterations = 0;
output.cgiterations =[];

%% get info
[~,nu]=size(B);
ny=size(C,1);
u0=f(1:nu);
y=f(nu+1:nu+ny);

xkk=xkk1+M*(y-C*xkk1);  % kalman

%% solver
p=[f(1:nu);xkk;f(ny+nu+1:2*ny+nu)];

b=S*p+s;
h=F*p;
tic
[zopt,~,~,output]=quadprog(H,h,G,b,[],[],[],[],[],options); % solve the optimal control problem
%[zopt,time,~] = wgsSolver(H,h,-G,-b,[],[],[],[],[],2);
time = toc;
feasRes=G*zopt-b;
iter = output.iterations;

nu=length(u0);
u=zopt(1:nu)+u0;

xk1k=A*xkk1+B*u+L*(y-C*xkk1); % kalman
